simulink model "gb_lqr_ia_npc_2017a"  (R2017a)
settings: Solver=FixedStepAuto  StartTime=0.0  StopTime=60  FixedStep=Ts  RelTol=1e-3  EnableMultiTasking=on
InitFcn:
  | run('../setup.m');
  | run('../model.m');
  | run('controller_ia.m')
values from neighbouring files (symbols this model uses):
  K1 = lqrd(A1i, B1i, C1i'*C1i, 0.01, Ts)    [controller_ia.m]
  K2 = A2(2,2)^2/(4*B2(2,1))    [controller_ia.m]
undefined symbols (not defined in the file or in its folder): a, ag, alpha, beta, C1, C2, Cg, Cm, DiscIntNeverNeededParam, g, Jphi, Jpsi, Jw, L, m, M, R, T, Ts, W
libraries: simulink_extras x6, legoev3lib x5, simulink x3, shared_linuxserviceslib x1
settings Model: ExtModeTrigDuration=2  Creator=thh206  LastModifiedBy=thh206
settings SolverCC: PositivePriorityOrder=on
settings OptimizationCC: EnhancedBackFolding=on  PassReuseOutputArgsAs=Individual arguments  MaxStackSize=64  OptimizeBlockOrder=speed
settings DebuggingCC: ParameterTunabilityLossMsg=error
settings HardwareCC: ProdBitPerPointer=32  ProdBitPerSizeT=32  ProdBitPerPtrDiffT=32  ProdLargestAtomicInteger=Long  ProdWordSize=32  ProdHWDeviceType=ARM Compatible->ARM 9
settings SFSimCC: MATLABDynamicMemAlloc=off
settings RTWCC: SystemTargetFile=ert.tlc  HardwareBoard=LEGO MINDSTORMS EV3  TLCOptions="-aInlineSetEventsForThisBaseRateFcn=TLC_FALSE -aSuppressMultiTaskScheduler=TLC_FALSE  -aRateBasedStepFcn=0"  TemplateMakefile=ert_default_tmf  Description=Embedded Coder  GenerateReport=on  Toolchain=Sourcery G++ Lite v2009q3  IncludeHyperlinkInReport=on  LaunchReport=on  GenerateTraceInfo=on  GenerateTraceReport=on  GenerateTraceReportSl=on  GenerateTraceReportSf=on  GenerateTraceReportEml=on
settings CodeAppCC: ForceParamTrailComments=on  IgnoreCustomStorageClasses=off  OperatorAnnotations=on  SimulinkDataObjDesc=on  SFDataObjDesc=on  InsertBlockDesc=on
settings ERTTargetCC: SupportContinuousTime=on  SupportVariableSizeSignals=on

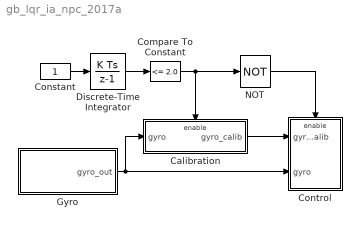
== system gb_lqr_ia_npc_2017a ==
  Calibration : Subsystem
  Compare To Constant : simulink/Logic and Bit Operations/Compare To Constant  relop=<=  const=2.0  OutDataTypeStr=boolean
  Constant : Constant
  Control : Subsystem
  Discrete-Time Integrator : DiscreteIntegrator  InitialConditionSetting=State (most efficient)  SampleTime=Ts  ICPrevOutput=DiscIntNeverNeededParam  ICPrevScaledInput=DiscIntNeverNeededParam
  Gyro : Subsystem  Variant=on  VariantControl=Variant1
  NOT : Logic  Operator=NOT  IconShape=distinctive  AllPortsSameDT=off  OutDataTypeStr=boolean
  wires:
  Gyro/1(" gyro_out") -> Calibration/1(gyro), Control/2(gyro)
  Discrete-Time Integrator/1 -> Compare To Constant/1
  Compare To Constant/1 -> Calibration/Enable, NOT/1
  Constant/1 -> Discrete-Time Integrator/1
  NOT/1 -> Control/Enable
  Calibration/1(gyro_calib) -> Control/1(gyro_calib)

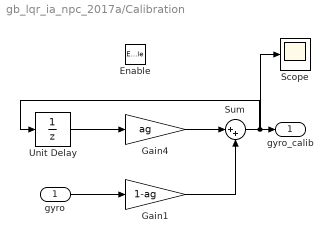
== system gb_lqr_ia_npc_2017a/Calibration ==
  gyro : Inport
  Enable : EnablePort
  Gain1 : Gain  Gain=1-ag  OutDataTypeStr=Inherit: Same as input  ParamDataTypeStr=Inherit: Same as input
  Gain4 : Gain  Gain=ag  OutDataTypeStr=Inherit: Same as input  ParamDataTypeStr=Inherit: Same as input
  Scope : Scope
  Sum : Sum  Inputs=|++  OutDataTypeStr=Inherit: Same as first input
  Unit Delay : UnitDelay  InitialCondition=[0]  SampleTime=Ts  HasFrameUpgradeWarning=on
  gyro_calib : Outport
  wires:
  Unit Delay/1 -> Gain4/1
  Gain4/1 -> Sum/1
  Gain1/1 -> Sum/2
  Sum/1 -> Scope/1, gyro_calib/1, Unit Delay/1
  gyro/1 -> Gain1/1

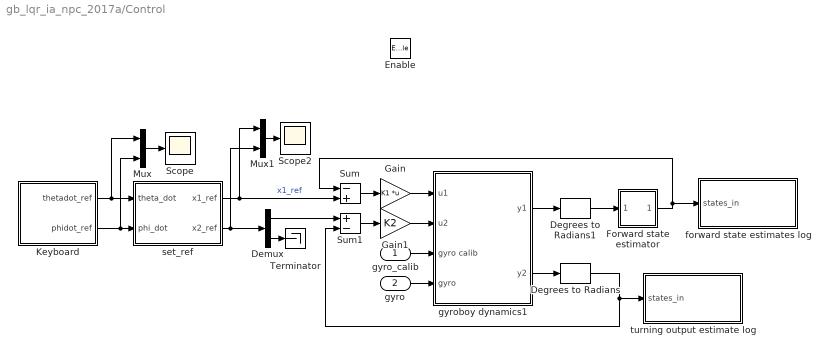
== system gb_lqr_ia_npc_2017a/Control ==
  gyro_calib : Inport
  gyro : Inport  Port=2
  Enable : EnablePort
  Degrees to Radians : simulink_extras/Transformations/Degrees to Radians
  Degrees to Radians1 : simulink_extras/Transformations/Degrees to Radians
  Demux : Demux  Outputs=2
  Forward state estimator : Subsystem
  Gain : Gain  Gain=K1  Multiplication=Matrix(K*u)
  Gain1 : Gain  Gain=K2
  Keyboard : Subsystem
  Mux : Mux  Inputs=2
  Mux1 : Mux  Inputs=2
  Scope : Scope
  Scope2 : Scope
  Sum : Sum  Inputs=-+
  Sum1 : Sum  Inputs=+-
  Terminator : Terminator
  forward state estimates log : Subsystem  Variant=on  VariantControl=Variant1
  gyroboy dynamics1 : Subsystem  Variant=on  VariantControl=Variant1
  set_ref : Subsystem
  turning output estimate log : Subsystem  Variant=on  VariantControl=Variant1
  wires:
  Keyboard/2(phidot_ref) -> Mux/2, set_ref/2(phi_dot)
  Keyboard/1(thetadot_ref) -> Mux/1, set_ref/1(theta_dot)
  Degrees to Radians/1 -> turning output estimate log/1(states_in), Sum1/2
  Gain/1 -> gyroboy dynamics1/1(u1)
  Gain1/1 -> gyroboy dynamics1/2(u2)
  Sum1/1 -> Gain1/1
  gyroboy dynamics1/2(y2) -> Degrees to Radians/1
  Mux/1 -> Scope/1
  Degrees to Radians1/1 -> Forward state estimator/1(y1)
  gyroboy dynamics1/1(y1) -> Degrees to Radians1/1
  Demux/1 -> Sum1/1
  Sum/1 -> Gain/1
  Forward state estimator/1(x1e) -> forward state estimates log/1(states_in), Sum/1
  Demux/2 -> Terminator/1
  set_ref/1(x1_ref) -> Sum/2, Mux1/1  "x1_ref"
  gyro_calib/1 -> gyroboy dynamics1/3(gyro calib)
  gyro/1 -> gyroboy dynamics1/4(gyro)
  set_ref/2(x2_ref) -> Mux1/2, Demux/1
  Mux1/1 -> Scope2/1

== system gb_lqr_ia_npc_2017a/Gyro ==
  EV3 : Subsystem  VariantControl=EV3 == 1
  Simulation : Subsystem  VariantControl=(default)
  " gyro_out" : Outport

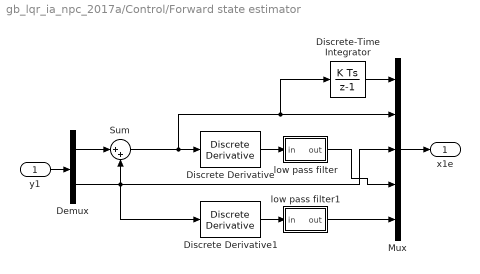
== system gb_lqr_ia_npc_2017a/Control/Forward state estimator ==
  y1 : Inport
  Demux : Demux  Outputs=2
  Discrete Derivative : simulink/Discrete/Discrete Derivative  gainval=1.0  ICPrevScaledInput=0.0  OutMin=[]  OutMax=[]  OutDataType=fixdt(1, 16)  OutScaling=2^-10  DoSatur=off
  Discrete Derivative1 : simulink/Discrete/Discrete Derivative  gainval=1.0  ICPrevScaledInput=0.0  OutMin=[]  OutMax=[]  OutDataType=fixdt(1, 16)  OutScaling=2^-10  DoSatur=off
  Discrete-Time Integrator : DiscreteIntegrator  InitialConditionSetting=State (most efficient)  SampleTime=-1  ICPrevOutput=DiscIntNeverNeededParam  ICPrevScaledInput=DiscIntNeverNeededParam
  Mux : Mux  Inputs=5
  Sum : Sum  Inputs=|++
  low pass filter : Subsystem
  low pass filter1 : Subsystem
  x1e : Outport
  wires:
  Sum/1 -> Discrete-Time Integrator/1, Mux/2, Discrete Derivative/1
  Demux/2 -> Mux/3, Discrete Derivative1/1, Sum/2
  Mux/1 -> x1e/1
  Demux/1 -> Sum/1
  y1/1 -> Demux/1
  Discrete Derivative/1 -> low pass filter/1(in)
  Discrete Derivative1/1 -> low pass filter1/1(in)
  low pass filter/1(out) -> Mux/4
  low pass filter1/1(out) -> Mux/5
  Discrete-Time Integrator/1 -> Mux/1

== system gb_lqr_ia_npc_2017a/Control/Keyboard ==
  Demux1 : Demux  Outputs=2
  MATLAB Function1 : MATLAB Function  TreatAsAtomicUnit=on
  Scope1 : Scope
  Unit Delay2 : UnitDelay  InitialCondition=[1;1]  SampleTime=-1  HasFrameUpgradeWarning=on
  Unit Delay3 : UnitDelay  InitialCondition=[0;0]  SampleTime=-1  HasFrameUpgradeWarning=on
  keyboard_control : Subsystem  Variant=on  VariantControl=Variant1
  thetadot_ref : Outport
  phidot_ref : Outport  Port=2
  wires:
  Demux1/1 -> thetadot_ref/1
  MATLAB Function1/1(y) -> Unit Delay3/1, Demux1/1
  Unit Delay3/1 -> MATLAB Function1/2(yp)
  MATLAB Function1/2(x) -> Unit Delay2/1
  Unit Delay2/1 -> MATLAB Function1/3(xp)
  Demux1/2 -> phidot_ref/1
  keyboard_control/1(keyboard) -> MATLAB Function1/1(u), Scope1/1

== system gb_lqr_ia_npc_2017a/Control/forward state estimates log ==
  states_in : Inport
  EV3 : Subsystem  VariantControl=EV3 == 1
  Simulation : Subsystem  VariantControl=(default)

== system gb_lqr_ia_npc_2017a/Control/gyroboy dynamics1 ==
  u1 : Inport
  u2 : Inport  Port=2
  gyro calib : Inport  Port=3
  gyro : Inport  Port=4
  EV3 : Subsystem  VariantControl=EV3 == 1
  Simulation : Subsystem  VariantControl=(default)
  y1 : Outport
  y2 : Outport  Port=2

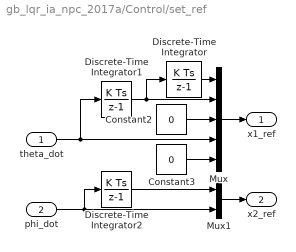
== system gb_lqr_ia_npc_2017a/Control/set_ref ==
  theta_dot : Inport
  phi_dot : Inport  Port=2
  Constant2 : Constant  Value=0
  Constant3 : Constant  Value=0
  Discrete-Time Integrator : DiscreteIntegrator  InitialConditionSetting=State (most efficient)  SampleTime=-1  ICPrevOutput=DiscIntNeverNeededParam  ICPrevScaledInput=DiscIntNeverNeededParam
  Discrete-Time Integrator1 : DiscreteIntegrator  InitialConditionSetting=State (most efficient)  SampleTime=-1  ICPrevOutput=DiscIntNeverNeededParam  ICPrevScaledInput=DiscIntNeverNeededParam
  Discrete-Time Integrator2 : DiscreteIntegrator  InitialConditionSetting=State (most efficient)  SampleTime=-1  ICPrevOutput=DiscIntNeverNeededParam  ICPrevScaledInput=DiscIntNeverNeededParam
  Mux : Mux  Inputs=5
  Mux1 : Mux  Inputs=2
  x1_ref : Outport
  x2_ref : Outport  Port=2
  wires:
  Constant2/1 -> Mux/3
  Constant3/1 -> Mux/5
  Mux/1 -> x1_ref/1
  Discrete-Time Integrator1/1 -> Discrete-Time Integrator/1, Mux/2
  phi_dot/1 -> Mux1/2, Discrete-Time Integrator2/1
  Discrete-Time Integrator2/1 -> Mux1/1
  theta_dot/1 -> Mux/4, Discrete-Time Integrator1/1
  Mux1/1 -> x2_ref/1
  Discrete-Time Integrator/1 -> Mux/1

== system gb_lqr_ia_npc_2017a/Control/turning output estimate log ==
  states_in : Inport
  EV3 : Subsystem  VariantControl=EV3 == 1
  Simulation : Subsystem  VariantControl=(default)

== system gb_lqr_ia_npc_2017a/Gyro/EV3 ==
  Data Type Conversion1 : DataTypeConversion  OutDataTypeStr=double
  Gain : Gain  Gain=-1
  Gyro Sensor : legoev3lib/Gyro Sensor  portNumber=2  sampleTime=Ts
      settings: SourceProductName=Simulink Support Package for LEGO MINDSTORMS EV3 Hardware  SourceProductBaseCode=LEGOEV3
  gyro_out : Outport
  wires:
  Gyro Sensor/1 -> Data Type Conversion1/1
  Data Type Conversion1/1 -> Gain/1
  Gain/1 -> gyro_out/1

== system gb_lqr_ia_npc_2017a/Gyro/Simulation ==
  Constant : Constant  Value=0.0
  gyro_out : Outport
  wires:
  Constant/1 -> gyro_out/1

== system gb_lqr_ia_npc_2017a/Control/Forward state estimator/low pass filter ==
  in : Inport
  Gain2 : Gain  Gain=a  OutDataTypeStr=Inherit: Same as input  ParamDataTypeStr=Inherit: Same as input
  Gain3 : Gain  Gain=1-a  OutDataTypeStr=Inherit: Same as input  ParamDataTypeStr=Inherit: Same as input
  Sum1 : Sum  Inputs=|++  OutDataTypeStr=Inherit: Same as first input
  Unit Delay : UnitDelay  SampleTime=-1  HasFrameUpgradeWarning=on
  out : Outport
  wires:
  Sum1/1 -> out/1, Unit Delay/1
  Gain3/1 -> Sum1/1
  Gain2/1 -> Sum1/2
  Unit Delay/1 -> Gain2/1
  in/1 -> Gain3/1

== system gb_lqr_ia_npc_2017a/Control/Forward state estimator/low pass filter1 ==
  in : Inport
  Gain2 : Gain  Gain=a  OutDataTypeStr=Inherit: Same as input  ParamDataTypeStr=Inherit: Same as input
  Gain3 : Gain  Gain=1-a  OutDataTypeStr=Inherit: Same as input  ParamDataTypeStr=Inherit: Same as input
  Sum1 : Sum  Inputs=|++  OutDataTypeStr=Inherit: Same as first input
  Unit Delay : UnitDelay  SampleTime=-1  HasFrameUpgradeWarning=on
  out : Outport
  wires:
  Sum1/1 -> out/1, Unit Delay/1
  Gain3/1 -> Sum1/1
  Gain2/1 -> Sum1/2
  Unit Delay/1 -> Gain2/1
  in/1 -> Gain3/1

== system gb_lqr_ia_npc_2017a/Control/Keyboard/keyboard_control ==
  EV3 : Subsystem  VariantControl=EV3 == 1
  Simulation : Subsystem  VariantControl=(default)
  keyboard : Outport

== system gb_lqr_ia_npc_2017a/Control/forward state estimates log/EV3 ==
  states_in : Inport
  Forward states estimates : Scope
  wires:
  states_in/1 -> Forward states estimates/1

== system gb_lqr_ia_npc_2017a/Control/forward state estimates log/Simulation ==
  states_in : Inport
  Forward states estimates : Scope
  wires:
  states_in/1 -> Forward states estimates/1

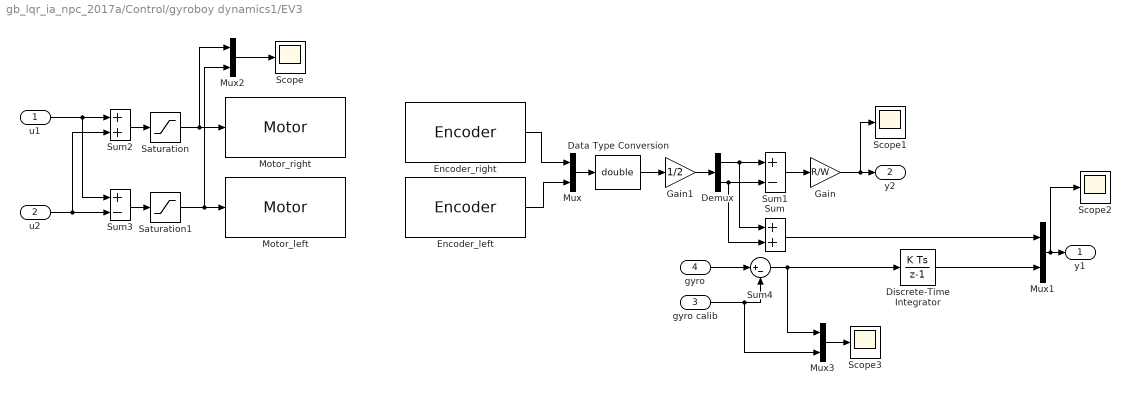
== system gb_lqr_ia_npc_2017a/Control/gyroboy dynamics1/EV3 ==
  u1 : Inport
  u2 : Inport  Port=2
  gyro calib : Inport  Port=3
  gyro : Inport  Port=4
  Data Type Conversion : DataTypeConversion  OutDataTypeStr=double
  Demux : Demux  Outputs=2
  Discrete-Time Integrator : DiscreteIntegrator  InitialConditionSetting=State (most efficient)  SampleTime=Ts  ICPrevOutput=DiscIntNeverNeededParam  ICPrevScaledInput=DiscIntNeverNeededParam
  Encoder_left : legoev3lib/Encoder  portNumber=D  opMode=No reset  sampleTime=Ts
      settings: SourceProductName=Simulink Support Package for LEGO MINDSTORMS EV3 Hardware  SourceProductBaseCode=LEGOEV3
  Encoder_right : legoev3lib/Encoder  portNumber=A  opMode=No reset  sampleTime=Ts
      settings: SourceProductName=Simulink Support Package for LEGO MINDSTORMS EV3 Hardware  SourceProductBaseCode=LEGOEV3
  Gain : Gain  Gain=R/W
  Gain1 : Gain  Gain=1/2
  Motor_left : legoev3lib/Motor  sportNumber=D  sstopAction=Brake
  Motor_right : legoev3lib/Motor  sportNumber=A  sstopAction=Brake
  Mux{,1..3} (4 alike) : Mux  Inputs=2
  Saturation : Saturate  UpperLimit=100  LowerLimit=-100
  Saturation1 : Saturate  UpperLimit=100  LowerLimit=-100
  Scope{,1..3} (4 alike) : Scope
  Sum : Sum
  Sum1 : Sum  Inputs=+-
  Sum2 : Sum
  Sum3 : Sum  Inputs=+-
  Sum4 : Sum  Inputs=|+-
  y1 : Outport
  y2 : Outport  Port=2
  wires:
  u1/1 -> Sum3/1, Sum2/1
  Saturation/1 -> Mux2/1, Motor_right/1
  u2/1 -> Sum2/2, Sum3/2
  Saturation1/1 -> Mux2/2, Motor_left/1
  Mux/1 -> Data Type Conversion/1
  Encoder_right/1 -> Mux/1
  Encoder_left/1 -> Mux/2
  Data Type Conversion/1 -> Gain1/1
  Gain1/1 -> Demux/1
  Demux/1 -> Sum/1, Sum1/1
  Demux/2 -> Sum/2, Sum1/2
  Sum/1 -> Mux1/1
  gyro/1 -> Sum4/1
  gyro calib/1 -> Mux3/2, Sum4/2
  Mux2/1 -> Scope/1
  Sum1/1 -> Gain/1
  Sum3/1 -> Saturation1/1
  Sum2/1 -> Saturation/1
  Discrete-Time Integrator/1 -> Mux1/2
  Sum4/1 -> Discrete-Time Integrator/1, Mux3/1
  Gain/1 -> Scope1/1, y2/1
  Mux1/1 -> Scope2/1, y1/1
  Mux3/1 -> Scope3/1

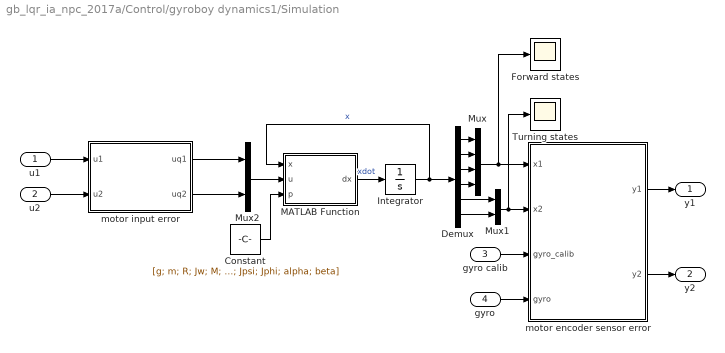
== system gb_lqr_ia_npc_2017a/Control/gyroboy dynamics1/Simulation ==
  u1 : Inport
  u2 : Inport  Port=2
  gyro calib : Inport  Port=3
  gyro : Inport  Port=4
  Constant : Constant  Value=[g; m; R; Jw; M; W; L; T; Jpsi; Jphi; alpha; beta]
  Demux : Demux  Outputs=6
  Forward states : Scope
  Integrator : Integrator  InitialCondition=[0;0;0;0;0;0]
  MATLAB Function : MATLAB Function  TreatAsAtomicUnit=on
  Mux : Mux
  Mux1 : Mux  Inputs=2
  Mux2 : Mux  Inputs=2
  Turning states : Scope
  motor encoder sensor error : Subsystem  Variant=on  VariantControl=Variant1
  motor input error : Subsystem  Variant=on  VariantControl=Variant1
  y1 : Outport
  y2 : Outport  Port=2
  wires:
  u1/1 -> motor input error/1("u1 ")
  u2/1 -> motor input error/2(u2)
  motor encoder sensor error/1(" y1") -> y1/1
  motor encoder sensor error/2(" y2") -> y2/1
  gyro calib/1 -> motor encoder sensor error/3(gyro_calib)
  gyro/1 -> motor encoder sensor error/4(gyro)
  MATLAB Function/1(dx) -> Integrator/1  "xdot"
  Integrator/1 -> MATLAB Function/1(x), Demux/1  "x"
  Demux/4 -> Mux/4
  Demux/3 -> Mux/3
  Demux/2 -> Mux/2
  Demux/1 -> Mux/1
  Demux/6 -> Mux1/2
  Demux/5 -> Mux1/1
  Mux/1 -> Forward states/1, motor encoder sensor error/1("x1 ")
  Mux1/1 -> Turning states/1, motor encoder sensor error/2(x2)
  motor input error/1(" uq1") -> Mux2/1
  motor input error/2(uq2) -> Mux2/2
  Mux2/1 -> MATLAB Function/2(u)
  Constant/1 -> MATLAB Function/3(p)

== system gb_lqr_ia_npc_2017a/Control/turning output estimate log/EV3 ==
  states_in : Inport
  Scope1 : Scope
  wires:
  states_in/1 -> Scope1/1

== system gb_lqr_ia_npc_2017a/Control/turning output estimate log/Simulation ==
  states_in : Inport
  Forward states estimates : Scope
  wires:
  states_in/1 -> Forward states estimates/1

== system gb_lqr_ia_npc_2017a/Control/Keyboard/keyboard_control/EV3 ==
  keyboard_or_preprog : Subsystem  Variant=on  VariantControl=Variant1
  keyboard : Outport
  wires:
  keyboard_or_preprog/1(keyboard) -> keyboard/1

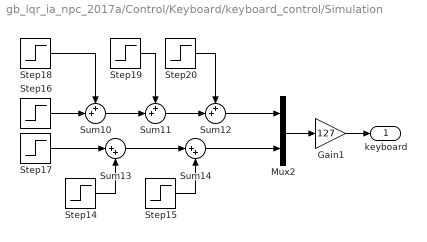
== system gb_lqr_ia_npc_2017a/Control/Keyboard/keyboard_control/Simulation ==
  Gain1 : Gain  Gain=127
  Mux2 : Mux  Inputs=2
  Step14 : Step  Time=46  After=-2  SampleTime=0
  Step15 : Step  Time=52  SampleTime=0
  Step16 : Step  Time=4  SampleTime=0
  Step17 : Step  Time=40  SampleTime=0
  Step18 : Step  Time=14  After=-1  SampleTime=0
  Step19 : Step  Time=24  After=-1  SampleTime=0
  Step20 : Step  Time=34  SampleTime=0
  Sum10 : Sum  Inputs=++|
  Sum11 : Sum  Inputs=++|
  Sum12 : Sum  Inputs=++|
  Sum13 : Sum  Inputs=|++
  Sum14 : Sum  Inputs=|++
  keyboard : Outport
  wires:
  Mux2/1 -> Gain1/1
  Gain1/1 -> keyboard/1
  Step15/1 -> Sum14/2
  Sum10/1 -> Sum11/2
  Sum13/1 -> Sum14/1
  Sum14/1 -> Mux2/2
  Step16/1 -> Sum10/2
  Sum11/1 -> Sum12/2
  Sum12/1 -> Mux2/1
  Step20/1 -> Sum12/1
  Step18/1 -> Sum10/1
  Step17/1 -> Sum13/1
  Step19/1 -> Sum11/1
  Step14/1 -> Sum13/2

== system gb_lqr_ia_npc_2017a/Control/gyroboy dynamics1/Simulation/motor encoder sensor error ==
  "x1 " : Inport
  x2 : Inport  Port=2
  gyro_calib : Inport  Port=3
  gyro : Inport  Port=4
  ideal sensors : Subsystem  VariantControl=(default)
  sensor quantisation and saturation : Subsystem  VariantControl=quant_sat == 1
  " y1" : Outport
  " y2" : Outport  Port=2

== system gb_lqr_ia_npc_2017a/Control/gyroboy dynamics1/Simulation/motor input error ==
  "u1 " : Inport
  u2 : Inport  Port=2
  ideal motor : Subsystem  VariantControl=(default)
  motor quantisation and saturation : Subsystem  VariantControl=quant_sat == 1
  " uq1" : Outport
  uq2 : Outport  Port=2

== system gb_lqr_ia_npc_2017a/Control/Keyboard/keyboard_control/EV3/keyboard_or_preprog ==
  kb_or_xb : Subsystem  VariantControl=preprog == 0
  preprog : Subsystem  VariantControl=(default)
  keyboard : Outport

== system gb_lqr_ia_npc_2017a/Control/gyroboy dynamics1/Simulation/motor encoder sensor error/ideal sensors ==
  "x1 " : Inport
  x2 : Inport  Port=2
  Gain : Gain  Gain=C1  Multiplication=Matrix(K*u)
  Gain1 : Gain  Gain=C2  Multiplication=Matrix(K*u)
  Radians to Degrees : simulink_extras/Transformations/Radians to Degrees
  Radians to Degrees1 : simulink_extras/Transformations/Radians to Degrees
  " y1" : Outport
  y2 : Outport  Port=2
  wires:
  "x1 "/1 -> Radians to Degrees/1
  Gain/1 -> " y1"/1
  x2/1 -> Radians to Degrees1/1
  Radians to Degrees/1 -> Gain/1
  Radians to Degrees1/1 -> Gain1/1
  Gain1/1 -> y2/1

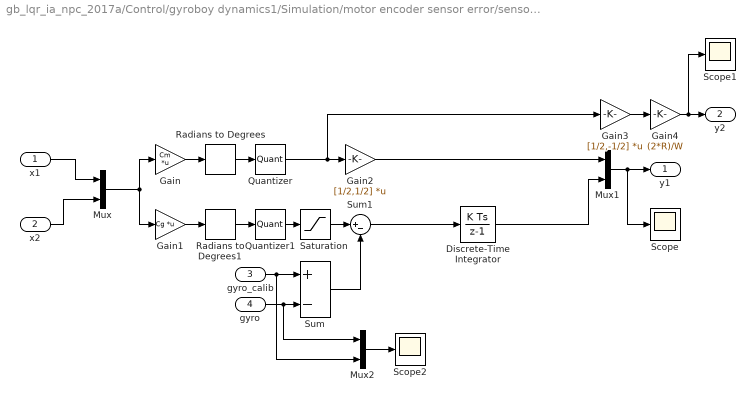
== system gb_lqr_ia_npc_2017a/Control/gyroboy dynamics1/Simulation/motor encoder sensor error/sensor quantisation and saturation ==
  "x1 " : Inport
  x2 : Inport  Port=2
  gyro_calib : Inport  Port=3
  gyro : Inport  Port=4
  Discrete-Time Integrator : DiscreteIntegrator  InitialConditionSetting=State (most efficient)  SampleTime=Ts  ICPrevOutput=DiscIntNeverNeededParam  ICPrevScaledInput=DiscIntNeverNeededParam
  Gain : Gain  Gain=Cm  Multiplication=Matrix(K*u)
  Gain1 : Gain  Gain=Cg  Multiplication=Matrix(K*u)
  Gain2 : Gain  Gain=[1/2,1/2]  Multiplication=Matrix(K*u)
  Gain3 : Gain  Gain=[1/2,-1/2]  Multiplication=Matrix(K*u)
  Gain4 : Gain  Gain=(2*R)/W
  Mux : Mux  Inputs=2
  Mux1 : Mux  Inputs=2
  Mux2 : Mux  Inputs=2
  Quantizer : Quantizer  QuantizationInterval=1
  Quantizer1 : Quantizer  QuantizationInterval=1
  Radians to Degrees : simulink_extras/Transformations/Radians to Degrees
  Radians to Degrees1 : simulink_extras/Transformations/Radians to Degrees
  Saturation : Saturate  UpperLimit=500  LowerLimit=-500
  Scope : Scope
  Scope1 : Scope
  Scope2 : Scope
  Sum : Sum  Inputs=+-
  Sum1 : Sum  Inputs=|+-
  " y1" : Outport
  y2 : Outport  Port=2
  wires:
  Quantizer1/1 -> Saturation/1
  "x1 "/1 -> Mux/1
  x2/1 -> Mux/2
  Radians to Degrees/1 -> Quantizer/1
  Mux/1 -> Gain1/1, Gain/1
  Gain1/1 -> Radians to Degrees1/1
  Quantizer/1 -> Gain3/1, Gain2/1
  Gain2/1 -> Mux1/1
  Gain/1 -> Radians to Degrees/1
  Radians to Degrees1/1 -> Quantizer1/1
  gyro_calib/1 -> Mux2/2, Sum/1
  gyro/1 -> Mux2/1, Sum/2
  Saturation/1 -> Sum1/1
  Sum/1 -> Sum1/2
  Mux1/1 -> Scope/1, " y1"/1
  Gain3/1 -> Gain4/1
  Gain4/1 -> Scope1/1, y2/1
  Sum1/1 -> Discrete-Time Integrator/1
  Discrete-Time Integrator/1 -> Mux1/2
  Mux2/1 -> Scope2/1

== system gb_lqr_ia_npc_2017a/Control/gyroboy dynamics1/Simulation/motor input error/ideal motor ==
  "u1 " : Inport
  u2 : Inport  Port=2
  " uq1" : Outport
  uq2 : Outport  Port=2
  wires:
  "u1 "/1 -> " uq1"/1
  u2/1 -> uq2/1

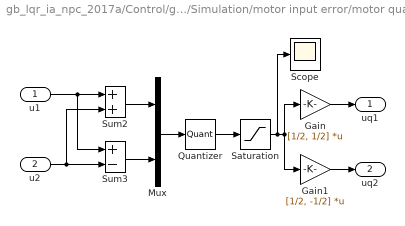
== system gb_lqr_ia_npc_2017a/Control/gyroboy dynamics1/Simulation/motor input error/motor quantisation and saturation ==
  "u1 " : Inport
  u2 : Inport  Port=2
  Gain : Gain  Gain=[1/2, 1/2]  Multiplication=Matrix(K*u)
  Gain1 : Gain  Gain=[1/2, -1/2]  Multiplication=Matrix(K*u)
  Mux : Mux  Inputs=2
  Quantizer : Quantizer  QuantizationInterval=1
  Saturation : Saturate  UpperLimit=100  LowerLimit=-100
  Scope : Scope
  Sum2 : Sum
  Sum3 : Sum  Inputs=+-
  " uq1" : Outport
  uq2 : Outport  Port=2
  wires:
  Saturation/1 -> Scope/1, Gain1/1, Gain/1
  Sum2/1 -> Mux/1
  u2/1 -> Sum2/2, Sum3/2
  Quantizer/1 -> Saturation/1
  Sum3/1 -> Mux/2
  Mux/1 -> Quantizer/1
  "u1 "/1 -> Sum3/1, Sum2/1
  Gain/1 -> " uq1"/1
  Gain1/1 -> uq2/1

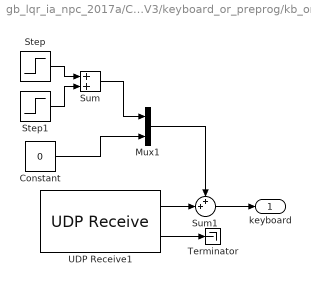
== system gb_lqr_ia_npc_2017a/Control/Keyboard/keyboard_control/EV3/keyboard_or_preprog/kb_or_xb ==
  Constant : Constant  Value=0
  Mux1 : Mux  Inputs=2
  Step : Step  Time=2.5  After=50  SampleTime=0
  Step1 : Step  Time=5.5  After=-50  SampleTime=0
  Sum : Sum
  Sum1 : Sum  Inputs=++|
  Terminator : Terminator
  UDP Receive1 : shared_linuxserviceslib/UDP Receive  localURL='0.0.0.0'  localPort=25000  remoteURL='0.0.0.0'  remotePort=-1  recvBufferSize=8192  signalDatatype=double  dims=2  isVarSize=off  showBlockingTime=off  blockingTime=0  sampletime=Ts  blockPlatform=LEGO EV3
  keyboard : Outport
  wires:
  UDP Receive1/2 -> Terminator/1
  Sum1/1 -> keyboard/1
  Mux1/1 -> Sum1/1
  Step1/1 -> Sum/2
  Constant/1 -> Mux1/2
  Sum/1 -> Mux1/1
  Step/1 -> Sum/1
  UDP Receive1/1 -> Sum1/2

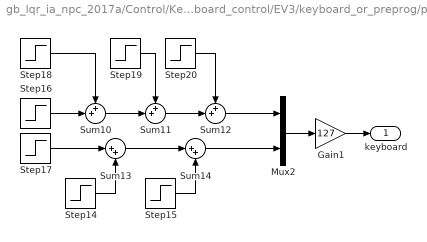
== system gb_lqr_ia_npc_2017a/Control/Keyboard/keyboard_control/EV3/keyboard_or_preprog/preprog ==
  Gain1 : Gain  Gain=127
  Mux2 : Mux  Inputs=2
  Step14 : Step  Time=46  After=-2  SampleTime=0
  Step15 : Step  Time=52  SampleTime=0
  Step16 : Step  Time=4  SampleTime=0
  Step17 : Step  Time=40  SampleTime=0
  Step18 : Step  Time=14  After=-1  SampleTime=0
  Step19 : Step  Time=24  After=-1  SampleTime=0
  Step20 : Step  Time=34  SampleTime=0
  Sum10 : Sum  Inputs=++|
  Sum11 : Sum  Inputs=++|
  Sum12 : Sum  Inputs=++|
  Sum13 : Sum  Inputs=|++
  Sum14 : Sum  Inputs=|++
  keyboard : Outport
  wires:
  Mux2/1 -> Gain1/1
  Gain1/1 -> keyboard/1
  Step15/1 -> Sum14/2
  Sum10/1 -> Sum11/2
  Sum13/1 -> Sum14/1
  Sum14/1 -> Mux2/2
  Step16/1 -> Sum10/2
  Sum11/1 -> Sum12/2
  Sum12/1 -> Mux2/1
  Step20/1 -> Sum12/1
  Step18/1 -> Sum10/1
  Step17/1 -> Sum13/1
  Step19/1 -> Sum11/1
  Step14/1 -> Sum13/2

== matlab function gb_lqr_ia_npc_2017a/Control/Keyboard/MATLAB Function1 ==
  data: u input; y output; yp input; xp input; x output
function [y,x] = fcn(u, yp, xp)
maxController = 127; % maximum controller input
u = u/maxController; % normalise inputs
x = xp; % this is an unused state of the robot to be used for collision avoidance
y = yp; % the current value of the reference signal
thetadotref = yp(1);
phidotref = yp(2);
acctheta = 4*0.002; %maximum increment in theta in one time step (0.002s)
thetadotmax = abs(6*u(1)); %maximum forward speed
phidotmax = 0.4*u(2); %increment in phi in one time step (0.002s)

% if up was pressed, accelerate
if abs(u(1)) > (15/maxController)
    if abs(thetadotref) <= thetadotmax
        thetadotref = thetadotref + acctheta*u(1);
    elseif thetadotref > thetadotmax
        thetadotref = thetadotref + acctheta*min(u(1),0);
    else 
        thetadotref = thetadotref + acctheta*max(u(1),0);
    end
else
    if thetadotref > acctheta/2
        thetadotref = thetadotref - acctheta;
    elseif thetadotref < -acctheta/2
        thetadotref = thetadotref + acctheta;
    else
        thetadotref = 0;
    end
end

% turning
if abs(u(2)) > (15/maxController)
    phidotref = -phidotmax;
else
    phidotref = 0;
end

y = [thetadotref; phidotref];
end

== matlab function gb_lqr_ia_npc_2017a/Control/gyroboy dynamics1/Simulation/MATLAB Function ==
  data: x input; u input; dx output; p input
function dx = fcn(x,u,p)
g = p(1); m = p(2); R = p(3); Jw = p(4); M = p(5); W = p(6); L = p(7);
T = p(8); Jpsi = p(9); Jphi = p(10); alpha = p(11); beta = p(12);

P = [(2*m+M)*R^2 + 2*Jw, M*L*R*cos(x(2)); M*L*R*cos(x(2)), M*L^2 + Jpsi];
Q = m*R^2 + 2*Jphi*R^2/(W^2) + Jw + 2*M*L^2*R^2*(sin(x(2)))^2/(W^2);
dx = [x(3);
    x(4);
    P\[M*L*R*x(4)^2*sin(x(2)) + 2*beta*x(4) - 2*beta*x(3) + 2*alpha*u(1);
    M*g*L*sin(x(2)) + M*L^2*(x(6)^2)*sin(x(2))*cos(x(2)) + 2*beta*(x(3)-x(4)) - 2*alpha*u(1)];
    x(6);
    ((2*R*alpha*u(2)/W) - (beta*x(6)) - (4*M*R^2*L^2*x(6)*x(4)*sin(x(2))*cos(x(2))/(W^2)))/Q];
end
